simulink model "LabC_CompensatorOverRobot"  (R2018b)
settings: Solver=FixedStepDiscrete  StartTime=0.0  StopTime=inf  FixedStep=fSamplingPeriod  RelTol=1e-3  EnableMultiTasking=on
values from neighbouring files (symbols this model uses):
  Cd = [1 0 0 0 ... (first row only)    [LabB_ObserverOverSimulator_Discrete_Parameters.m]    (also in LabC_CompensatorOverRobot_Parameters.m = [1 0 0 0])
  fGyroBias = -363    [GyroBias.mat]    (also in LabC_CompensatorOverRobot_Parameters.m = fGyroBias + 23)
  fGyroConversionFactor = -1/131    (= -0.00763358778626)    [LabB_ObserverAndControllerOverRobot_Parameters.m]    (also in LabC_CompensatorOverRobot_Parameters.m)
  fSamplingPeriod = 0.005    [FinalRun26_Robot_Data_Sampling_rt_200.mat]    (also in FinalRun27_Robot_Data_Sampling_rt_200.mat; FinalRun28_Robot_Data_Sampling_rt_200.mat; FinalRun29_Robot_Data_Sampling_rt_200.mat; GetDataFromSerial.m = 1/sampFreq)
  fWheelRadius = 0.0216    [LabB_ObserverAndControllerOverRobot_Parameters.m]    (also in LabC_CompensatorOverRobot_Parameters.m)
  iNumberOfEncoderSteps = 720    [LabB_ObserverAndControllerOverRobot_Parameters.m]    (also in LabC_CompensatorOverRobot_Parameters.m)
  Ld = Lt'    [LabB_ObserverOverSimulator_Discrete_Parameters.m]
  Md1 = Atxx-La*Atyx-Lna*Ctx    [LabB_ObserverOverSimulator_Discrete_Parameters.m]
  Md2 = Btx - La*Bty    [LabB_ObserverOverSimulator_Discrete_Parameters.m]
  Md3 = Atxy-La*Atyy-Lna*Cty    [LabB_ObserverOverSimulator_Discrete_Parameters.m]
  Md4 = Lna    [LabB_ObserverOverSimulator_Discrete_Parameters.m]
  Md5 = La    [LabB_ObserverOverSimulator_Discrete_Parameters.m]
  Md6 = T(:,1)    [LabB_ObserverOverSimulator_Discrete_Parameters.m]
  Md7 = T(:,2:end)    [LabB_ObserverOverSimulator_Discrete_Parameters.m]
  Nud = Nvec(end)    [LabC_CompensatorOverRobot_Parameters.m]
  Nxd = Nvec(1:r)    [LabC_CompensatorOverRobot_Parameters.m]
undefined symbols (not defined in the file or in its folder): Ad, Bd, DiscIntNeverNeededParam, Kd, sigbuilder_block
libraries: simulink x16, arduinolib x3, cstblocks x2
settings Model: FPTRunName=FPA_Reference  SimulationMode=external  ExtModeTrigDuration=2  Creator=Alec  LastModifiedBy=j
settings DataIOCC: SaveFormat=Array  SaveOutput=off  SignalLogging=off  DSMLogging=off  SaveTime=off
settings OptimizationCC: EnhancedBackFolding=on  PassReuseOutputArgsAs=Individual arguments  ExpressionDepthLimit=2147483647  MaxStackSize=64  OptimizeBlockOrder=speed  DifferentSizesBufferReuse=on  OptimizationCustomize=off
settings DebuggingCC: UnderspecifiedInitializationDetection=Classic  MergeDetectMultiDrivingBlocksExec=none  ParameterTunabilityLossMsg=error  StateNameClashWarn=warning  SFUnexpectedBacktrackingDiag=warning  SFNoUnconditionalDefaultTransitionDiag=warning  SFExecutionAtInitializationDiag=none
settings HardwareCC: ProdBitPerInt=16  ProdBitPerPointer=16  ProdBitPerSizeT=16  ProdBitPerPtrDiffT=16  ProdLargestAtomicFloat=None  ProdWordSize=8  ProdHWDeviceType=Atmel->AVR  UseEmbeddedCoderFeatures=off  UseSimulinkCoderFeatures=off
settings ModelReferenceCC: PropagateSignalLabelsOutOfModel=off
settings SFSimCC: SimUseLocalCustomCode=off  MATLABDynamicMemAlloc=off
settings RTWCC: SystemTargetFile=ert.tlc  HardwareBoard=Arduino Mega 2560  TemplateMakefile=ert_default_tmf  GenerateReport=on  RTWVerbose=off  RTWUseLocalCustomCode=off  Toolchain=Arduino AVR  BuildConfiguration=Faster Runs  IncludeHyperlinkInReport=on  LaunchReport=on  GenerateTraceInfo=on  GenerateTraceReport=on  GenerateTraceReportSl=on  GenerateTraceReportSf=on  GenerateTraceReportEml=on
settings CodeAppCC: ForceParamTrailComments=on  IgnoreCustomStorageClasses=off  OperatorAnnotations=on  SimulinkDataObjDesc=on  SFDataObjDesc=on  CustomSymbolStrType=$N$R$M  InsertBlockDesc=on  InternalIdentifier=Classic
settings ERTTargetCC: SupportContinuousTime=on  SupportNonInlinedSFcns=on  SupportVariableSizeSignals=on
settings ConfigComp: CovMetricSettings=dw  CovHtmlReporting=on  CovSaveCumulativeToWorkspaceVar=on  CovSaveSingleToWorkspaceVar=on  CovExternalEMLEnable=off

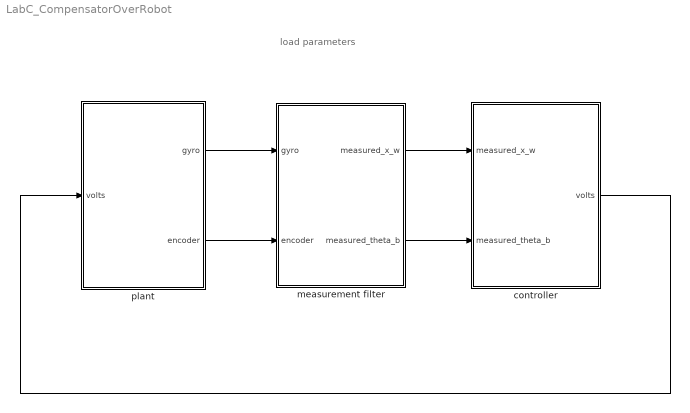
== system LabC_CompensatorOverRobot ==
  note: load parameters
  controller : Subsystem
  measurement filter : Subsystem
  plant : Subsystem
  wires:
  plant/1(gyro) -> measurement filter/1(gyro)
  measurement filter/2(measured_theta_b) -> controller/2("measured_theta_b ")
  measurement filter/1(measured_x_w) -> controller/1(measured_x_w)
  plant/2(encoder) -> measurement filter/2(encoder)
  controller/1(volts) -> plant/1(volts)

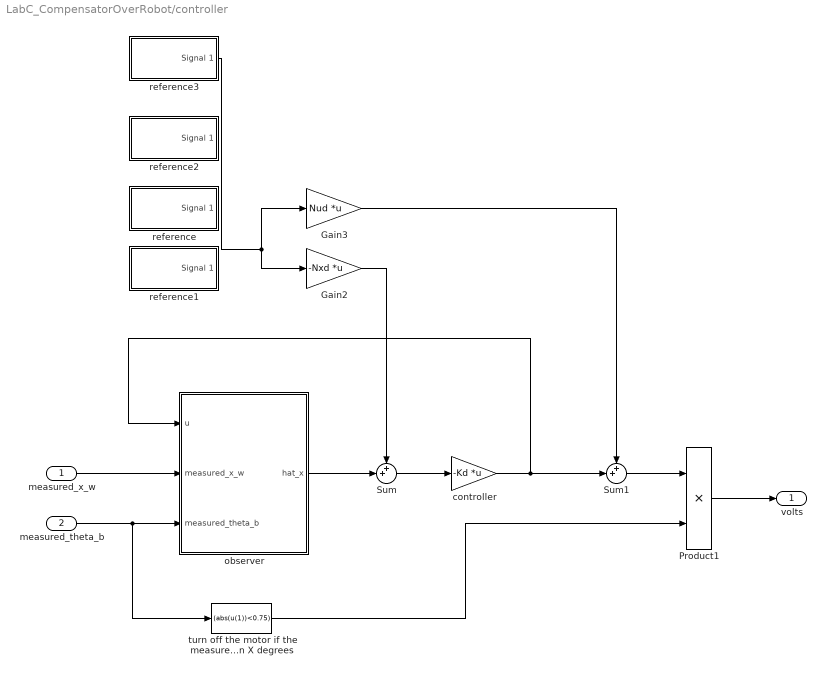
== system LabC_CompensatorOverRobot/controller ==
  measured_x_w : Inport
  "measured_theta_b " : Inport  Port=2
  Gain2 : Gain  Gain=-Nxd  Multiplication=Matrix(K*u)
  Gain3 : Gain  Gain=Nud  Multiplication=Matrix(K*u)
  Product1 : Product  RndMeth=Zero
  Sum : Sum  Inputs=++|
  Sum1 : Sum  Inputs=++|
  controller : Gain  Gain=-Kd  Multiplication=Matrix(K*u)
  observer : Subsystem
  reference : Subsystem  Tag=STV Subsys  LoadFcn=sigbuilder_block('load');  StartFcn=sigbuilder_block('start');  StopFcn=sigbuilder_block('stop');  ClipboardFcn=sigbuilder_block('clipboard');  mask(Sigbuilder block){tuvar=[0:10]}
      mask help: Simulink:masks:SigbuilderBlock_MD
      mask init:
      | if ~strcmp(get_param(bdroot(gcbh),'SimulationStatus'),'stopped') tuvar = sigbuilder_block('maskInit'); end
      settings: CopyFcn=sigbuilder_block('copy');  DeleteFcn=sigbuilder_block('delete');  ModelCloseFcn=sigbuilder_block('modelClose');  PreSaveFcn=sigbuilder_block('preSave');  PauseFcn=sigbuilder_block('pause');  ContinueFcn=sigbuilder_block('continue');  NameChangeFcn=sigbuilder_block('namechange');  OpenFcn=sigbuilder_block('open',[437.6 199.2 550.4 400 ]);  CloseFcn=sigbuilder_block('close');
      mask Display: plot(0, 0, 100, 100,[2, 2, 32, 32, 2], [68, 8, 8, 68, 68],[32, 2], [38, 38], [32, 19, 2],[53, 60, 44], [32, 17, 17, 2],[16, 16, 31, 31]);txt = getActiveGroup(gcbh);text(2, 100, txt,'verticalAlignment', 'top');
  reference1 : Subsystem  Tag=STV Subsys  LoadFcn=sigbuilder_block('load');  StartFcn=sigbuilder_block('start');  StopFcn=sigbuilder_block('stop');  ClipboardFcn=sigbuilder_block('clipboard');  mask(Sigbuilder block){tuvar=[0:10]}
      mask help: Simulink:masks:SigbuilderBlock_MD
      mask init:
      | if ~strcmp(get_param(bdroot(gcbh),'SimulationStatus'),'stopped') tuvar = sigbuilder_block('maskInit'); end
      settings: CopyFcn=sigbuilder_block('copy');  DeleteFcn=sigbuilder_block('delete');  ModelCloseFcn=sigbuilder_block('modelClose');  PreSaveFcn=sigbuilder_block('preSave');  PauseFcn=sigbuilder_block('pause');  ContinueFcn=sigbuilder_block('continue');  NameChangeFcn=sigbuilder_block('namechange');  OpenFcn=sigbuilder_block('open',[437.6 199.2 550.4 400 ]);  CloseFcn=sigbuilder_block('close');
      mask Display: plot(0, 0, 100, 100,[2, 2, 32, 32, 2], [68, 8, 8, 68, 68],[32, 2], [38, 38], [32, 19, 2],[53, 60, 44], [32, 17, 17, 2],[16, 16, 31, 31]);txt = getActiveGroup(gcbh);text(2, 100, txt,'verticalAlignment', 'top');
  reference2 : Subsystem  Tag=STV Subsys  LoadFcn=sigbuilder_block('load');  StartFcn=sigbuilder_block('start');  StopFcn=sigbuilder_block('stop');  ClipboardFcn=sigbuilder_block('clipboard');  mask(Sigbuilder block){tuvar=[0:10]}
      mask help: Simulink:masks:SigbuilderBlock_MD
      mask init:
      | if ~strcmp(get_param(bdroot(gcbh),'SimulationStatus'),'stopped') tuvar = sigbuilder_block('maskInit'); end
      settings: CopyFcn=sigbuilder_block('copy');  DeleteFcn=sigbuilder_block('delete');  ModelCloseFcn=sigbuilder_block('modelClose');  PreSaveFcn=sigbuilder_block('preSave');  PauseFcn=sigbuilder_block('pause');  ContinueFcn=sigbuilder_block('continue');  NameChangeFcn=sigbuilder_block('namechange');  OpenFcn=sigbuilder_block('open',[437.6 199.2 550.4 400 ]);  CloseFcn=sigbuilder_block('close');
      mask Display: plot(0, 0, 100, 100,[2, 2, 32, 32, 2], [68, 8, 8, 68, 68],[32, 2], [38, 38], [32, 19, 2],[53, 60, 44], [32, 17, 17, 2],[16, 16, 31, 31]);txt = getActiveGroup(gcbh);text(2, 100, txt,'verticalAlignment', 'top');
  reference3 : Subsystem  Tag=STV Subsys  LoadFcn=sigbuilder_block('load');  StartFcn=sigbuilder_block('start');  StopFcn=sigbuilder_block('stop');  ClipboardFcn=sigbuilder_block('clipboard');  mask(Sigbuilder block){tuvar=[0:10]}
      mask help: Simulink:masks:SigbuilderBlock_MD
      mask init:
      | if ~strcmp(get_param(bdroot(gcbh),'SimulationStatus'),'stopped') tuvar = sigbuilder_block('maskInit'); end
      settings: CopyFcn=sigbuilder_block('copy');  DeleteFcn=sigbuilder_block('delete');  ModelCloseFcn=sigbuilder_block('modelClose');  PreSaveFcn=sigbuilder_block('preSave');  PauseFcn=sigbuilder_block('pause');  ContinueFcn=sigbuilder_block('continue');  NameChangeFcn=sigbuilder_block('namechange');  OpenFcn=sigbuilder_block('open',[437.6 199.2 550.4 400 ]);  CloseFcn=sigbuilder_block('close');
      mask Display: plot(0, 0, 100, 100,[2, 2, 32, 32, 2], [68, 8, 8, 68, 68],[32, 2], [38, 38], [32, 19, 2],[53, 60, 44], [32, 17, 17, 2],[16, 16, 31, 31]);txt = getActiveGroup(gcbh);text(2, 100, txt,'verticalAlignment', 'top');
  turn off the motor if the measured angle is greater than X degrees : Fcn  Expr=(abs(u(1))<0.75)
  volts : Outport
  wires:
  observer/1(hat_x) -> Sum/2
  turn off the motor if the measured angle is greater than X degrees/1 -> Product1/2
  "measured_theta_b "/1 -> observer/3(measured_theta_b), turn off the motor if the measured angle is greater than X degrees/1
  controller/1 -> Sum1/2, observer/1(u)
  measured_x_w/1 -> observer/2(measured_x_w)
  Product1/1 -> volts/1
  Sum/1 -> controller/1
  Sum1/1 -> Product1/1
  Gain2/1 -> Sum/1
  Gain3/1 -> Sum1/1
  reference3/1(Signal 1) -> Gain3/1, Gain2/1

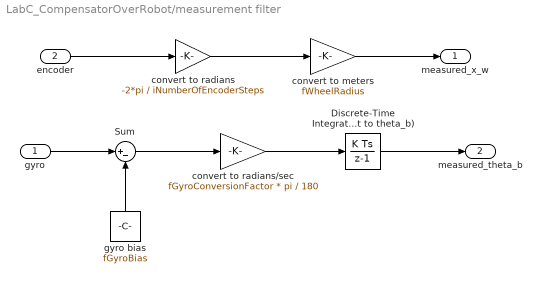
== system LabC_CompensatorOverRobot/measurement filter ==
  gyro : Inport
  encoder : Inport  Port=2
  Discrete-Time Integrator (convert from theta_b_dot to theta_b) : DiscreteIntegrator  SampleTime=fSamplingPeriod  OutDataTypeStr=Inherit: Inherit via back propagation  ICPrevOutput=DiscIntNeverNeededParam  ICPrevScaledInput=DiscIntNeverNeededParam
  Sum : Sum  Inputs=|+-
  convert to radians/sec : Gain  Gain=fGyroConversionFactor * pi / 180  OutDataTypeStr=Inherit: Same as input
  convert to radians : Gain  Gain=-2*pi / iNumberOfEncoderSteps  OutDataTypeStr=Inherit: Same as input
  convert to meters : Gain  Gain=fWheelRadius  OutDataTypeStr=Inherit: Same as input
  gyro bias : Constant  Value=fGyroBias  OutDataTypeStr=single
  measured_x_w : Outport
  measured_theta_b : Outport  Port=2
  wires:
  convert to radians/sec/1 -> Discrete-Time Integrator (convert from theta_b_dot to theta_b)/1
  gyro/1 -> Sum/1
  Sum/1 -> convert to radians/sec/1
  convert to radians/1 -> convert to meters/1
  encoder/1 -> convert to radians/1
  Discrete-Time Integrator (convert from theta_b_dot to theta_b)/1 -> measured_theta_b/1
  gyro bias/1 -> Sum/2
  convert to meters/1 -> measured_x_w/1

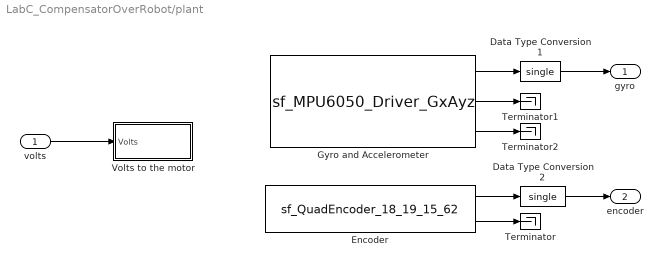
== system LabC_CompensatorOverRobot/plant ==
  volts : Inport
  Data Type Conversion1 : DataTypeConversion  OutDataTypeStr=single
  Data Type Conversion2 : DataTypeConversion  OutDataTypeStr=single
  "Encoder " : S-Function  InitFcn=try, set_param(gcb,'FunctionName','sf_QuadEncoder_18_19_15_62'), end  FunctionName=sf_QuadEncoder_18_19_15_62  Parameters=uint8([0 1]),uint8([18 62]),uint8([19 15])  SFunctionModules=sf_QuadEncoder_18_19_15_62_wrapper  SFunctionDeploymentMode=off  EnableBusSupport=off  mask(S-Function Builder){}
      mask init:
      | val = [[.9  0.75 0.75 1 1 .9 .9 1]',[1 1 0.75 0.75 .9 .9 1 .9]'];try , sys = get_param(gcb,'SfunBuilderFcnName');if isempty(sys), sys = get_param(gcb,'FunctionName'); end,catch, sys = get_param(gcb,'FunctionName'); end
      settings: CopyFcn=set_param(gcbh,'LinkStatus','none')  PreSaveFcn=try, set_param(gcb,'FunctionName','sf_QuadEncoder_18_19_15_62'), end  OpenFcn=sfunctionwizard(gcbh)
      mask Display: plot(val(:,1),val(:,2)),disp(sys), port_label('output',1,'pos1'), port_label('output',2,'pos2')
  Gyro and Accelerometer : S-Function  InitFcn=try, set_param(gcb,'FunctionName','sf_MPU6050_Driver_GxAyz'), end  FunctionName=sf_MPU6050_Driver_GxAyz  SFunctionModules=sf_MPU6050_Driver_GxAyz_wrapper  SFunctionDeploymentMode=off  EnableBusSupport=off  mask(S-Function Builder){}
      mask help: Simulink:masks:SFunctionBuilder_MD
      mask init: same as LabC_CompensatorOverRobot/plant/Encoder 
      settings: CopyFcn=set_param(gcbh,'LinkStatus','none')  PreSaveFcn=try, set_param(gcb,'FunctionName','sf_MPU6050_Driver_GxAyz'), end  OpenFcn=sfunctionwizard(gcbh)
      mask Display: plot(val(:,1),val(:,2)),disp(sys), port_label('output',1,'x_vel'), port_label('output',2,'y_acc'), port_label('output',3,'z_acc')
  Terminator : Terminator
  Terminator1 : Terminator
  Terminator2 : Terminator
  Volts to the motor : Subsystem
  gyro : Outport
  encoder : Outport  Port=2
  wires:
  Gyro and Accelerometer/1 -> Data Type Conversion1/1
  Data Type Conversion1/1 -> gyro/1
  "Encoder "/1 -> Data Type Conversion2/1
  Data Type Conversion2/1 -> encoder/1
  "Encoder "/2 -> Terminator/1
  Gyro and Accelerometer/2 -> Terminator1/1
  Gyro and Accelerometer/3 -> Terminator2/1
  volts/1 -> Volts to the motor/1(Volts)

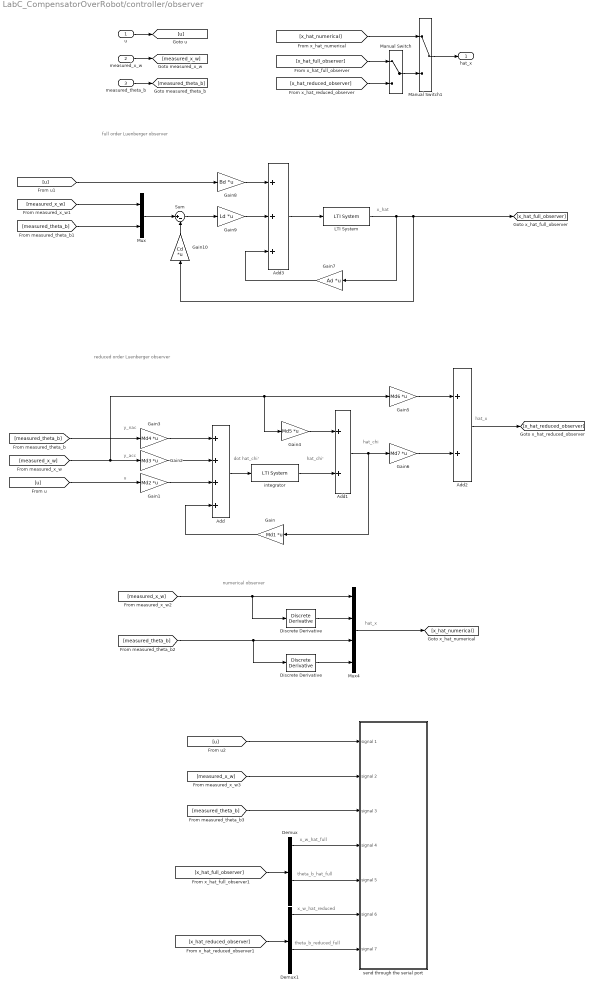
== system LabC_CompensatorOverRobot/controller/observer ==
  note: x_w_hat_full
  note: full order Luenberger observer
  note: reduced order Luenberger observer
  note: numerical observer
  note: hat_x
  note: hat_chi
  note: u
  note: dot hat_chi'
  note: hat_chi'
  note: y_acc
  note: y_nac
  note: x_hat
  note: hat_x
  note: x_w_hat_reduced
  note: theta_b_hat_full
  note: theta_b_reduced_full
  u : Inport
  measured_x_w : Inport  Port=2
  measured_theta_b : Inport  Port=3
  Add : Sum  Inputs=++++
  Add1 : Sum
  Add2 : Sum
  Add3 : Sum  Inputs=+++
  Demux : Demux
  Demux1 : Demux
  Discrete Derivative : simulink/Discrete/Discrete Derivative  gainval=1.0  ICPrevScaledInput=0.0  OutMin=[]  OutMax=[]  OutDataType=fixdt(1, 16)  OutScaling=2^-10  DoSatur=off
  "Discrete Derivative " : simulink/Discrete/Discrete Derivative  gainval=1.0  ICPrevScaledInput=0.0  OutMin=[]  OutMax=[]  OutDataType=fixdt(1, 16)  OutScaling=2^-10  DoSatur=off
  Gain : Gain  Gain=Md1  Multiplication=Matrix(K*u)
  Gain1 : Gain  Gain=Md2  Multiplication=Matrix(K*u)
  Gain10 : Gain  Gain=Cd  Multiplication=Matrix(K*u)
  Gain2 : Gain  Gain=Md3  Multiplication=Matrix(K*u)
  Gain3 : Gain  Gain=Md4  Multiplication=Matrix(K*u)
  Gain4 : Gain  Gain=Md5  Multiplication=Matrix(K*u)
  Gain5 : Gain  Gain=Md6  Multiplication=Matrix(K*u)
  Gain6 : Gain  Gain=Md7  Multiplication=Matrix(K*u)
  Gain7 : Gain  Gain=Ad  Multiplication=Matrix(K*u)
  Gain8 : Gain  Gain=Bd  Multiplication=Matrix(K*u)
  Gain9 : Gain  Gain=Ld  Multiplication=Matrix(K*u)
  LTI System : cstblocks/LTI System  sys=tf(1,[1 0],fSamplingPeriod)*eye(size(Ad))  IC=[]
  Manual Switch : ManualSwitch
  Manual Switch1 : ManualSwitch
  Mux : Mux  Inputs=2
  Mux4 : Mux
  Sum : Sum  Inputs=|+-
  integrator : cstblocks/LTI System  sys=tf(1,[1 0],fSamplingPeriod)*eye(3)  IC=[]
  send through the serial port : Subsystem
  hat_x : Outport
  wires:
  Gain3/1 -> Add/1
  Gain2/1 -> Add/2
  Add/1 -> integrator/1
  Gain4/1 -> Add1/1
  Gain1/1 -> Add/3
  Gain/1 -> Add/4
  integrator/1 -> Add1/2
  Add1/1 -> Gain/1, Gain6/1
  Gain5/1 -> Add2/1
  Gain6/1 -> Add2/2
  Discrete Derivative/1 -> Mux4/2
  "Discrete Derivative "/1 -> Mux4/4
  [measured_x_w] -> Gain4/1, Gain5/1, Gain2/1
  [measured_theta_b] -> Gain3/1
  Gain9/1 -> Add3/2
  Sum/1 -> Gain9/1
  [u] -> Gain1/1
  Gain8/1 -> Add3/1
  Gain10/1 -> Sum/2
  Mux/1 -> Sum/1
  Gain7/1 -> Add3/3
  LTI System/1 -> [x_hat_full_observer], Gain10/1, Gain7/1
  Add3/1 -> LTI System/1
  u/1 -> [u]
  measured_x_w/1 -> [measured_x_w]
  measured_theta_b/1 -> [measured_theta_b]
  [u] -> Gain8/1
  [measured_x_w] -> Mux/1
  [measured_theta_b] -> Mux/2
  [measured_x_w] -> Discrete Derivative/1, Mux4/1
  [measured_theta_b] -> "Discrete Derivative "/1, Mux4/3
  [u] -> send through the serial port/1(signal 1)
  [measured_x_w] -> send through the serial port/2(signal 2)
  [measured_theta_b] -> send through the serial port/3(signal 3)
  Mux4/1 -> [x_hat_numerical]
  [x_hat_full_observer] -> Manual Switch/1
  Manual Switch/1 -> Manual Switch1/2
  Manual Switch1/1 -> hat_x/1
  Add2/1 -> [x_hat_reduced_observer]
  [x_hat_reduced_observer] -> Manual Switch/2
  [x_hat_numerical] -> Manual Switch1/1
  [x_hat_full_observer] -> Demux/1
  Demux/1 -> send through the serial port/4(signal 4)
  Demux/3 -> send through the serial port/5(signal 5)
  Demux1/3 -> send through the serial port/7(signal 7)
  Demux1/1 -> send through the serial port/6(signal 6)
  [x_hat_reduced_observer] -> Demux1/1

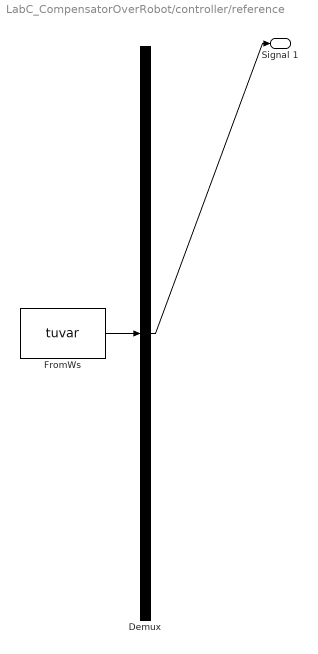
== system LabC_CompensatorOverRobot/controller/reference ==
  Demux : Demux  Tag=STV Demux  Outputs=1
  FromWs : FromWorkspace  Tag=STV FromWs  VariableName=tuvar  SampleTime=0  OutputAfterFinalValue=Holding final value
      SigBuilderData=|
      | common.afterFinalStr = 'Hold final value'
      | common.sampleTime = '0'
      | dataSet.timeRange = [0 30]
      | dataSet.name = 'Group 1'
      | sbobj.Groups.Name = 'Group 1'
      | sbobj.Groups.Signals.Name = 'Signal 1'
      | sbobj.Groups.Signals.XData = [0 10 14 30]
      | sbobj.Groups.Signals.YData = [0 0 0.6 0]
      | sbobj.Groups.TimeRange = [0 30]
  Signal 1 : Outport  Tag=STV Outport
  wires:
  FromWs/1 -> Demux/1
  Demux/1 -> Signal 1/1

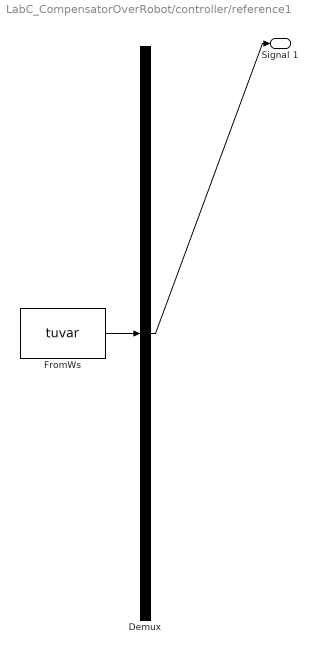
== system LabC_CompensatorOverRobot/controller/reference1 ==
  Demux : Demux  Tag=STV Demux  Outputs=1
  FromWs : FromWorkspace  Tag=STV FromWs  VariableName=tuvar  SampleTime=0  OutputAfterFinalValue=Holding final value
      SigBuilderData=|
      | common.afterFinalStr = 'Hold final value'
      | common.sampleTime = '0'
      | dataSet.timeRange = [0 30]
      | dataSet.name = 'Group 1'
      | sbobj.Groups.Name = 'Group 1'
      | sbobj.Groups.Signals.Name = 'Signal 1'
      | sbobj.Groups.Signals.XData = [0 10 20 30]
      | sbobj.Groups.Signals.YData = [0 0 2 2]
      | sbobj.Groups.TimeRange = [0 30]
  Signal 1 : Outport  Tag=STV Outport
  wires:
  FromWs/1 -> Demux/1
  Demux/1 -> Signal 1/1

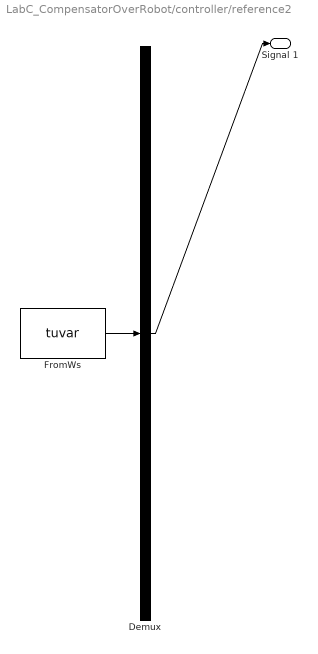
== system LabC_CompensatorOverRobot/controller/reference2 ==
  Demux : Demux  Tag=STV Demux  Outputs=1
  FromWs : FromWorkspace  Tag=STV FromWs  VariableName=tuvar  SampleTime=0  OutputAfterFinalValue=Holding final value
      SigBuilderData=|
      | common.afterFinalStr = 'Hold final value'
      | common.sampleTime = '0'
      | dataSet.timeRange = [0 60]
      | dataSet.name = 'Group 1'
      | sbobj.Groups.Name = 'Group 1'
      | sbobj.Groups.Signals.Name = 'Signal 1'
      | sbobj.Groups.Signals.XData = [0 0.5 1 1.5 2 2.5 3 3.5 4 4.5 5 5.5 6 6.5 7 7.5 8 8.5 9 9.5 10 10.5 11 11.5 12 12.5 13 13.5 14 14.5 15 15.5 16 16.5 17 17.5 18 18.5 19 19.5 20 20.5 21 21.5 22 22.5 23 23.5 24 24.5 25 25.5 26 26.5 27 27.5 28 28.5 29 29.5 30 30.5 31 31.5 32 32.5 33 33.5 34 34.5 35 35.5 36 36.5 37 37.5 38 38.5 39 39.5 40 40.5 41 41.5 42 42.5 43 43.5 44 44.5 45 45.5 46 46.5 47 47.5 48 48.5 49 49.5 50 50.5 51 51.5 52 52.5 53 53.5 54 54.5 55 55.5 56 56.5 57 57.5 58 58.5 59 59.5 60]
      | sbobj.Groups.Signals.YData = [0 0.0927050983125 0.176335575688 0.242705098312 0.285316954889 0.3 0.285316954889 0.242705098312 0.176335575688 0.0927050983125 1.69966166929e-16 -0.0927050983125 -0.176335575688 -0.242705098312 -0.285316954889 -0.3 -0.285316954889 -0.242705098312 -0.176335575688 -0.0927050983125 0 0.0927050983125 0.176335575688 0.242705098312 0.285316954889 0.3 0.285316954889 0.242705098312 0.176335575688 0.0927050983125 1.69966166929e-16 -0.0927050983125 -0.176335575688 -0.242705098312 -0.285316954889 -0.3 -0.285316954889 -0.242705098312 -0.176335575688 -0.0927050983125 0 0.0927050983125 0.176335575688 0.242705098312 0.285316954889 0.3 0.285316954889 0.242705098312 0.176335575688 0.0927050983125 1.69966166929e-16 -0.0927050983125 -0.176335575688 -0.242705098312 -0.285316954889 -0.3 -0.285316954889 -0.242705098312 -0.176335575688 -0.0927050983125 0 0.0927050983125 0.176335575688 0.242705098312 0.285316954889 0.3 0.285316954889 0.242705098312 0.176335575688 0.0927050983125 1.69966166929e-16 -0.0927050983125 -0.176335575688 -0.242705098312 -0.285316954889 -0.3 -0.285316954889 -0.242705098312 -0.176335575688 -0.0927050983125 0 0.0927050983125 0.176335575688 0.242705098312 0.285316954889 0.3 0.285316954889 0.242705098312 0.176335575688 0.0927050983125 1.69966166929e-16 -0.0927050983125 -0.176335575688 -0.242705098312 -0.285316954889 -0.3 -0.285316954889 -0.242705098312 -0.176335575688 -0.0927050983125 0 0.0927050983125 0.176335575688 0.242705098312 0.285316954889 0.3 0.285316954889 0.242705098312 0.176335575688 0.0927050983125 1.69966166929e-16 -0.0927050983125 -0.176335575688 -0.242705098312 -0.285316954889 -0.3 -0.285316954889 -0.242705098312 -0.176335575688 -0.0927050983125 0]
      | sbobj.Groups.TimeRange = [0 60]
  Signal 1 : Outport  Tag=STV Outport
  wires:
  FromWs/1 -> Demux/1
  Demux/1 -> Signal 1/1

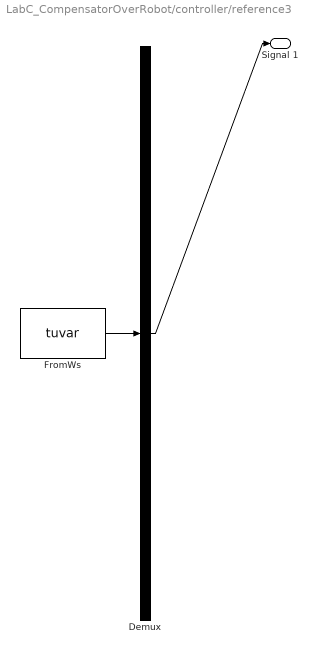
== system LabC_CompensatorOverRobot/controller/reference3 ==
  Demux : Demux  Tag=STV Demux  Outputs=1
  FromWs : FromWorkspace  Tag=STV FromWs  VariableName=tuvar  SampleTime=0  OutputAfterFinalValue=Holding final value
      SigBuilderData=|
      | common.afterFinalStr = 'Hold final value'
      | common.sampleTime = '0'
      | dataSet.timeRange = [0 60]
      | dataSet.name = 'Group 1'
      | sbobj.Groups.Name = 'Group 1'
      | sbobj.Groups.Signals.Name = 'Signal 1'
      | sbobj.Groups.Signals.XData = [0 60]
      | sbobj.Groups.Signals.YData = [0 0]
      | sbobj.Groups.TimeRange = [0 60]
  Signal 1 : Outport  Tag=STV Outport
  wires:
  FromWs/1 -> Demux/1
  Demux/1 -> Signal 1/1

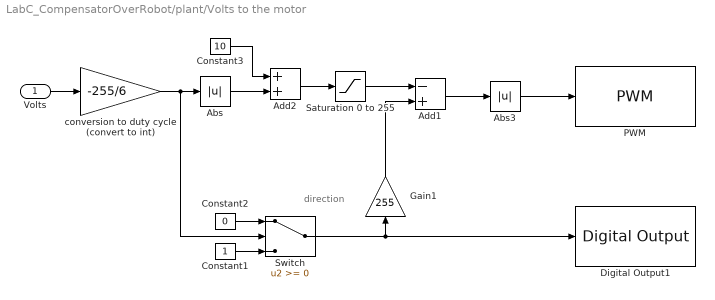
== system LabC_CompensatorOverRobot/plant/Volts to the motor ==
  note: direction
  Volts : Inport
  Abs : Abs
  Abs3 : Abs
  Add1 : Sum  Inputs=-+
  Add2 : Sum
  Constant1 : Constant
  Constant2 : Constant  Value=0
  Constant3 : Constant  Value=10
  Digital Output1 : arduinolib/Digital Output  pinNumber=6  blockPlatform=arduino
  Gain1 : Gain  Gain=255
  PWM : arduinolib/PWM  pinNumber=8  EnableInputFrequency=off  InitialFrequency=2000  InitialDutyCycle=0  NotificationType=None  blockPlatform=arduino
  Saturation 0 to 255 : Saturate  UpperLimit=255  LowerLimit=0
  Switch : Switch
  conversion to duty cycle (convert to int) : Gain  Gain=-255/6  OutDataTypeStr=int16
  wires:
  Volts/1 -> conversion to duty cycle (convert to int)/1
  Switch/1 -> Digital Output1/1, Gain1/1
  Constant2/1 -> Switch/1
  Constant1/1 -> Switch/3
  Gain1/1 -> Add1/2
  Add1/1 -> Abs3/1
  conversion to duty cycle (convert to int)/1 -> Switch/2, Abs/1
  Saturation 0 to 255/1 -> Add1/1
  Abs3/1 -> PWM/1
  Constant3/1 -> Add2/1
  Abs/1 -> Add2/2
  Add2/1 -> Saturation 0 to 255/1

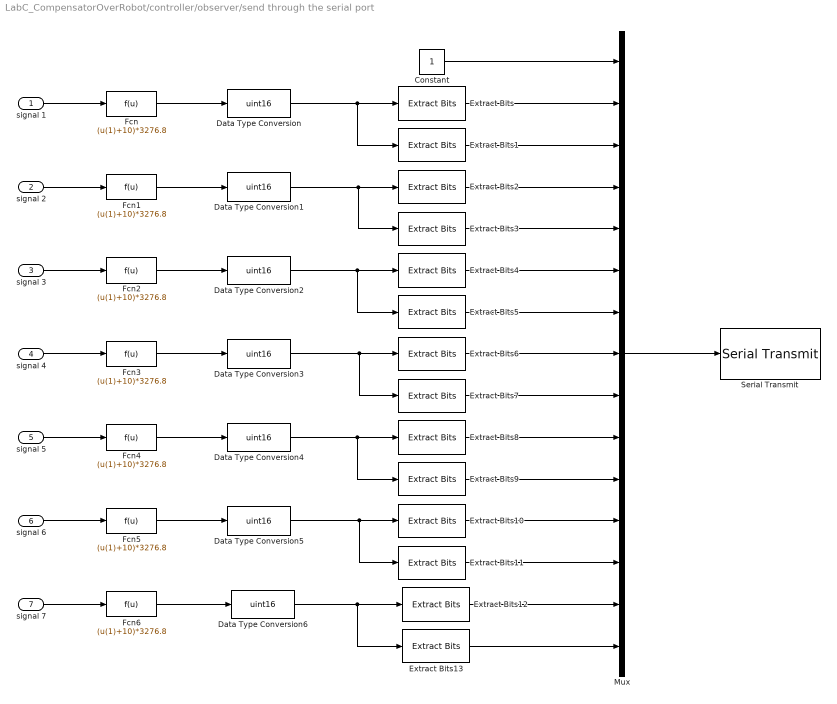
== system LabC_CompensatorOverRobot/controller/observer/send through the serial port ==
  signal 1 : Inport
  signal 2 : Inport  Port=2
  signal 3 : Inport  Port=3
  signal 4 : Inport  Port=4
  signal 5 : Inport  Port=5
  signal 6 : Inport  Port=6
  signal 7 : Inport  Port=7
  Constant : Constant  OutDataTypeStr=uint8
  Data Type Conversion{,1..6} (7 alike) : DataTypeConversion  OutDataTypeStr=uint16
  Extract Bits{,2,4,6,8,10,12} (7 alike) : simulink/Logic and Bit Operations/Extract Bits  bitsToExtract=Upper half  numBits=8  bitIdxRange=[0 7]  outScalingMode=Treat bit field as an integer
      settings: SourceProductName=Simulink
  Extract Bits{1,3,5,7,9,11,13} (7 alike) : simulink/Logic and Bit Operations/Extract Bits  bitsToExtract=Lower half  numBits=8  bitIdxRange=[0 7]  outScalingMode=Treat bit field as an integer
      settings: SourceProductName=Simulink
  Fcn{,1..6} (7 alike) : Fcn  Expr=(u(1)+10)*3276.8
  Mux : Mux  Inputs=15
  Serial Transmit : arduinolib/Serial Transmit  portNumber=0  sendmode=write  sendformat=Decimal  floatprecision=2  blockPlatform=arduino
      settings: SourceProductName=Simulink Support Package for Arduino Hardware
  wires:
  Data Type Conversion/1 -> Extract Bits1/1, Extract Bits/1
  Extract Bits/1 -> Mux/2
  Fcn1/1 -> Data Type Conversion1/1
  Fcn/1 -> Data Type Conversion/1
  Extract Bits2/1 -> Mux/4
  Constant/1 -> Mux/1
  Data Type Conversion1/1 -> Extract Bits2/1, Extract Bits3/1
  Extract Bits1/1 -> Mux/3
  Mux/1 -> Serial Transmit/1
  Extract Bits3/1 -> Mux/5
  Data Type Conversion3/1 -> Extract Bits6/1, Extract Bits7/1
  Extract Bits4/1 -> Mux/6
  Data Type Conversion2/1 -> Extract Bits5/1, Extract Bits4/1
  Extract Bits5/1 -> Mux/7
  Extract Bits6/1 -> Mux/8
  Fcn3/1 -> Data Type Conversion3/1
  Extract Bits7/1 -> Mux/9
  Fcn2/1 -> Data Type Conversion2/1
  Data Type Conversion4/1 -> Extract Bits9/1, Extract Bits8/1
  Fcn5/1 -> Data Type Conversion5/1
  Extract Bits8/1 -> Mux/10
  Extract Bits9/1 -> Mux/11
  Data Type Conversion5/1 -> Extract Bits10/1, Extract Bits11/1
  Extract Bits11/1 -> Mux/13
  Extract Bits10/1 -> Mux/12
  Fcn4/1 -> Data Type Conversion4/1
  signal 2/1 -> Fcn1/1
  signal 7/1 -> Fcn6/1
  signal 6/1 -> Fcn5/1
  signal 3/1 -> Fcn2/1
  signal 1/1 -> Fcn/1
  signal 4/1 -> Fcn3/1
  signal 5/1 -> Fcn4/1
  Extract Bits13/1 -> Mux/15
  Extract Bits12/1 -> Mux/14
  Fcn6/1 -> Data Type Conversion6/1
  Data Type Conversion6/1 -> Extract Bits12/1, Extract Bits13/1
